simulink model "BESS_Harness"  (R2025b)
settings: Solver=VariableStepAuto  StartTime=0.0  StopTime=5  RelTol=1e-3
PostLoadFcn:
  | BESSParam
values from neighbouring files (symbols this model uses):
  bessVoltage = 1500    [BESSGFLParam.m]    (also in BESSGFMParam.m)
  gflInverter = struct    [BESSGFLParam.m]
  gfmInverter = struct    [BESSGFMParam.m]
  Ts = 5E-5    (= 5e-05)    [BESSGFLParam.m]    (also in BESSGFMParam.m; WindFarmParam.m)
undefined symbols (not defined in the file or in its folder): bessSystem, DiscIntNeverNeededParam, solar
libraries: eeGeneralControl x26, nesl_utility x26, ee_lib x16, simulink x12, fl_lib x10, eeTransforms x7, nesl_utility_internal x4, slpidlib x2, batteryecm_lib x2, simulink_extras x1, eePowerMeasurement x1, eePwmGenerator x1
(part 1 of 4)
settings Model: SimulationMode=accelerator  Creator=skota  LastModifiedBy=skota

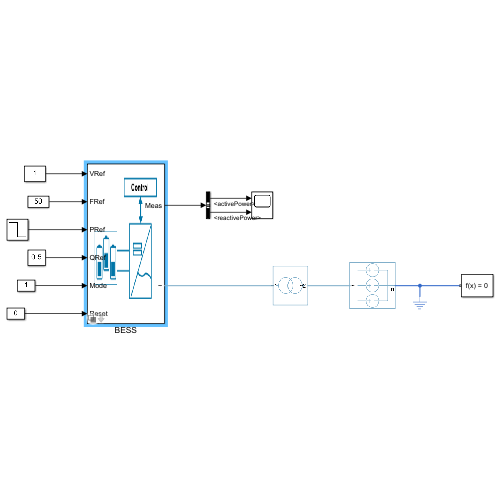
[thumbnail: Simulink's stored preview of the top-level diagram]
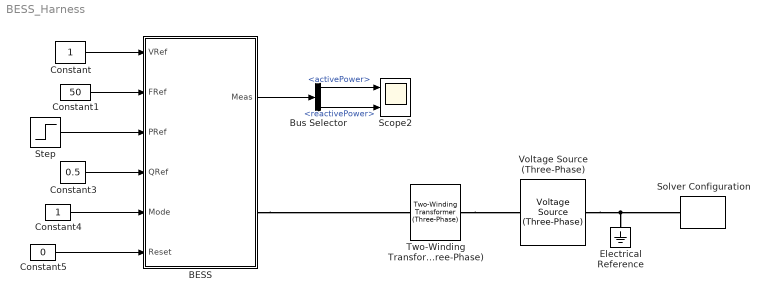
== system BESS_Harness ==
  BESS : Subsystem  Variant=on  VariantControlMode=label  LabelModeActiveChoice=Detailed  mask(Battery Energy Storage System (BESS)){fidelity=Detailed, bessController=Grid Forming, plantRating=bessSystem.plantRating, Vac=bessSystem.Vac, frequency=bessSystem.frequency, iMaxPU=bessSystem.iMaxPU, efficiency=bessSystem.converterEfficiency, baseVoltageDC=bessSystem.Vdc, filterInductance=bessSystem.filterInductance, filterResistance=bessSystem.filterResistance, maxSOC=bessSystem.maxSOC, minSOC=bessSystem.minSOC, converterFidelity=Average, fSw=bessSystem.switchingFrequency, activeDroop=bessSystem.activeDroop, reactiveDroop=bessSystem.reactiveDroop, maxSOCGFM=0.95, minSOCGFM=0.1, initialSOC=0.9, capacityType=Infinite, capacity=1000}
      mask prompts: fidelity "Modeling Option"; bessController "Operating Mode"; plantRating "BESS Rating (kW)"; Vac "Rated AC side voltage (phase-phase RMS) (V)"; frequency "Rated electrical frequency at AC side (Hz)"; iMaxPU "Maximum converter current (pu)"; efficiency "Converter Efficiency (%)"; baseVoltageDC "Voltage on DC side (V)"; filterInductance "Filter inductance (H)"; filterResistance "Filter series resistance (Ohm)"; maxSOC "Maximum  operating SOC"; minSOC "Minimum  operating SOC"; converterFidelity "Converter Fidelity"; fSw "Switching Frequency (kHz)"; activeDroop "Active droop"; reactiveDroop "Reactive droop"; maxSOCGFM "Maximum  operating SOC"; minSOCGFM "Minimum  operating SOC"; initialSOC "Initial SOC"; capacityType "Battery charge capacity"; capacity "Battery capacity (Ah)"
      mask help:
      | This block represents a flexible BESS that can be configured for different operational modes and modeling fidelities. It supports Grid-Following (GFL) and Grid-Forming (GFM) control strategies, along with two fidelity levels:
      |
      | Detailed – captures dynamic control loops and converter behavior for accurate transient analysis.
      | Simplified – optimized for faster simulations while preserving essential system characteristics.
      settings: CopyFcn=set_param(gcbh,'LinkStatus','none');
      mask Help: web('BESS.html')
      mask TypeOptions fidelity: Detailed | Simplified
      mask Callback fidelity:
      | component.mask.fidelitySelection;
      |     fidelity = get_param(gcb,'fidelity');
      |     mode = get_param(gcb,'bessController');
      |     maskObj = Simulink.Mask.get(gcb);
      |     allNames = {maskObj.Parameters.Name};
      |     effIdx = find(strcmp(allNames, 'efficiency'));
      |     tabGFL = maskObj.getDialogControl('cellSimplified');
      |     tabGFM = maskObj.getDialogControl('cellSimplifiedGFM');
      |     if strcmp(fidelity,'Simplified')
      |         maskObj.Parameters(effIdx).Visible = 'on';
      |         if strcmp(mode,'Grid Following')
      |             tabGFL.Visible = 'on';
      |             tabGFM.Visible = 'off';
      |         else
      |             tabGFL.Visible = 'off';
      |             tabGFM.Visible = 'on';
      |         end
      |     else
      |         maskObj.Parameters(effIdx).Visible = 'off';
      |         tabGFL.Visible = 'off';
      |         tabGFM.Visible = 'off';
      |     end
      mask TypeOptions bessController: Grid Following | Grid Forming
      mask Callback bessController:
      | fidelity = get_param(gcb,'fidelity');
      | mode = get_param(gcb,'bessController');
      | if strcmp(fidelity,'Detailed')
      |     component.mask.setBESSController;
      | else
      |     blockPath = [gcb,'/','Simplified'];
      |     component.mask.setBESSController(blockPath);
      | end
      | maskObj = Simulink.Mask.get(gcb);
      | tabGFL = maskObj.getDialogControl('cellSimplified');
      | tabGFM = maskObj.getDialogControl('cellSimplifiedGFM');
      | if strcmp(fidelity,'Simplified')
      |     if strcmp(mode,'Grid Following')
      |         tabGFL.Visible = 'on';
      |         tabGFM.Visible = 'off';
      |     else
      |         tabGFL.Visible = 'off';
      |         tabGFM.Visible = 'on';
      |     end
      | else
      |     tabGFL.Visible = 'off';
      |     tabGFM.Visible = 'off';
      | end
      mask TypeOptions converterFidelity: Detailed/BESS Plant/converterFidelity
      mask Callback converterFidelity:
      | blockPath = [gcb,'/','Detailed','/','BESS Plant','/','Converter'];
      | component.mask.converterFidelity(blockPath);
      mask TypeOptions fSw: Detailed/PV Plant & Controller/PV Plant/fSw
      mask TypeOptions initialSOC: Simplified/Grid Forming/initialSOC
      mask TypeOptions capacityType: Simplified/Grid Forming/capacityType
      mask Callback capacityType: component.mask.configureBatteryCapacity;
      mask TypeOptions capacity: Simplified/Grid Forming/capacity
      mask DialogControl generalDetailed Prompt: General
      mask DialogControl cellDetailed Prompt: Battery
      mask DialogControl configureBattery Prompt: Edit battery parameters
      mask DialogControl configureBattery Callback:
      | blockPath = [gcb,'/','Detailed','/','BESS Plant','/','Battery'] ;
      |     component.mask.openBlock(blockPath);
      mask DialogControl controllerDetailed Prompt: BESS Controller
      mask DialogControl configureBESSController Prompt: Edit BESS Controller
      mask DialogControl configureBESSController Callback:
      | controllerType = get_param(gcb,'bessController');
      |     blockPath = [gcb,'/','Detailed','/','BESS Controller','/',controllerType];
      |     component.mask.openBlock(blockPath);
      mask DialogControl cellSimplified Prompt: Battery
      mask DialogControl configureBatterySimplified Prompt: Edit battery parameters
      mask DialogControl configureBatterySimplified Callback:
      | mode = get_param(gcb,'bessController');
      |     blockPath = [gcb,'/','Simplified','/',mode,'/','Battery'] ;
      |     if strcmp(mode,'Grid Following')
      |         component.mask.openBlock(blockPath);
      |     end
      mask DialogControl converter Prompt: Converter
      mask DialogControl editConverter Prompt: Edit converter parameters
      mask DialogControl editConverter Callback:
      | converterFidelity = get_param(gcb,'converterFidelity');
      | blockPath = [gcb,'/','Detailed','/','BESS Plant','/','Converter','/',converterFidelity,'/','Converter'];
      | component.mask.openBlock(blockPath);
      mask DialogControl cellSimplifiedGFM Prompt: Battery
      mask Display: image('battery_detailed.png');
  Bus Selector : BusSelector  OutputSignals=activePower,reactivePower
  Constant : Constant
  Constant1 : Constant  Value=50
  Constant3 : Constant  Value=0.5
  Constant4 : Constant
  Constant5 : Constant  Value=0
  Electrical Reference : fl_lib/Electrical/Electrical Elements/Electrical Reference
  Scope2 : Scope  NumInputPorts=2
      settings: ActiveDisplayYMinimum=-3.20005915874359  ActiveDisplayYMaximum=1.7817477651289169  DataLoggingVariableName=ScopeData17
  Solver Configuration : nesl_utility/Solver Configuration  PhysicalDomain=network_engine_domain  SubClassName=solver  LeftPortType=input  RightPortType=generic  Tones=[]  Harmonics=[]  SimulateNoise=off  Profile=off  UseLocalSampling=off  EnableSwitchedLinearOptims=on  FrequencyDomain=off  UseCCode=off  RelTol=0.001  AbsTol=0.001  MinStep=1e-09  ToWorkspace=off  RevertToSquareIcSolve=off  NumHomotopyIterations=100  PhasorMode=off  PhasorModeNumHarmonics=1  ConsistencySolver=NEWTON_XTOL_AFTER_FTOL  IndexReductionMethod=DerivativeReplacement  DoDC=off  ResidualTolerance=1e-09  ConsistencyTolSource=GLOBAL  ConsistencyAbsTol=0.001  ConsistencyRelTol=0.001  ConsistencyTolFactor=1e3  UseLocalSolver=on  LocalSolverChoice=NE_BACKWARD_EULER_ADVANCER  ResolveIndetEquations=off  FunctionEvalNumThread=1  LocalSolverSampleTime=5e-5  DoFixedCost=on  MaxNonlinIter=1  MaxModeIter=2  ComputeImpulses=off  ImpulseIterations=2  LinearAlgebra=Sparse  LinearAlgebraNumThread=0  EquationFormulation=NE_TIME_EF  DelaysMemoryBudget=1024  AutomaticFiltering=off  FilteringTimeConstant=0.001  PartitionStorageMethod=AS_NEEDED  PartitionMemoryBudget=1024  PartitionMethod=ROBUST  MultibodyUseLocalSolver=off  MultibodyLocalSolverChoice=ODE1  MultibodyLocalSolverSampleTime=0.001
  Step : Step  Time=30  Before=1  After=0  SampleTime=0
  Two-Winding Transformer (Three-Phase) : ee_lib/Passive/Transformers/Two-Winding Transformer (Three-Phase)  SRated=200e6 A*V  FRated=50 Hz  Winding1Connection=ee.enum.windingconnection.Yg  VRated1=690 V  Winding2Connection=ee.enum.windingconnection.Yg  VRated2=6600 V  CoreType=ee.enum.coretype.threelimb  pu_Rw1=0.01  pu_Rw2=0.01  leakage_reactance_option=ee.enum.transformer_leakage.include  pu_Xl1=0.05  pu_Xl2=0.05  magnetizing_resistance_option=ee.enum.transformer_magnetizingResistance.exclude  pu_Rm=500  magnetizing_reactance_option=ee.enum.transformer_magnetizingReactance.exclude  saturation_option=ee.enum.transformer_saturation.exclude  pu_Xm=500  current_data=[0, .002, 1, 2]  magnetic_flux_data=[0, 1.2, 1.5, 1.51]  pu_X0=0.5  i1_specify=off  i1_priority=None  i1=[0, 0, 0] A  i1_nominal_specify=off  i1_nominal_value=1  i1_nominal_unit=A  i2_specify=off  i2_priority=None  i2=[0, 0, 0] A  i2_nominal_specify=off  i2_nominal_value=1  i2_nominal_unit=A  phi_specify=off  phi_priority=None  phi=[0, 0, 0]  phi_nominal_specify=off  phi_nominal_value=1  phi_nominal_unit=1  power_dissipated_specify=off  power_dissipated_priority=None  power_dissipated=0 W  power_dissipated_nominal_specify=off  power_dissipated_nominal_value=1  power_dissipated_nominal_unit=W
      settings: InternalSimscapePortConfiguration="{\"Bottom\":[],\"Left\":[{\"id\":\"N1\",\"label\":\"~1\",\"type\":\"foundation.electrical.three_phase\"}],\"Right\":[{\"id\":\"N2\",\"label\":\"~2\",\"type\":\"foundation.electrical.three_phase\"}],\"Top\":[]}"
  Voltage Source (Three-Phase) : ee_lib/Sources/Voltage Source (Three-Phase)  vline_rms=6600 V  shift=0 deg  freq=50 Hz  impedance_option=0  SShortCircuit=10e6 A*V  XR=15  R=0.01 Ohm  L=3.97e-4 H  harmonic_option=0  harmonic_orders=[5, 7, 11, 13]  harmonic_ratios=[.1, .1, .1, .1]  G_parasitic=0 1/Ohm  I_specify=off  I_priority=None  I=[0, 0, 0] A  I_nominal_specify=off  I_nominal_value=1  I_nominal_unit=A
  wires:
  Constant/1 -> BESS/1(VRef)
  Constant1/1 -> BESS/2(FRef)
  Constant3/1 -> BESS/4(QRef)
  Constant4/1 -> BESS/5(Mode)
  Constant5/1 -> BESS/6(Reset)
  Step/1 -> BESS/3(PRef)
  BESS/1(Meas) -> Bus Selector/1
  Bus Selector/1 -> Scope2/1  "<activePower>"
  Bus Selector/2 -> Scope2/2  "<reactivePower>"
  connections:
  BESS/RConn1 -- Two-Winding Transformer (Three-Phase)/LConn1
  Two-Winding Transformer (Three-Phase)/RConn1 -- Voltage Source (Three-Phase)/RConn1
  Voltage Source (Three-Phase)/LConn1 -- Solver Configuration/RConn1 -- Electrical Reference/LConn1

== system BESS_Harness/BESS ==
  VRef : Inport
  FRef : Inport  Port=2
  PRef : Inport  Port=3
  QRef : Inport  Port=4
  Mode : Inport  Port=5
  Reset : Inport  Port=6
  Detailed : Subsystem  VariantControl=Detailed
  Simplified : Subsystem  Variant=on  VariantControlMode=label  VariantControl=Simplified  LabelModeActiveChoice=Grid Forming
  ~ : PMIOPort  Side=Right
  Meas : Outport

== system BESS_Harness/BESS/Detailed ==
  note: Plant
  note: Controller
  VRef : Inport
  FRef : Inport  Port=2
  PRef : Inport  Port=3
  QRef : Inport  Port=4
  Mode : Inport  Port=5
  Reset : Inport  Port=6
  BESS Controller : Subsystem  Variant=on  VariantControlMode=label  LabelModeActiveChoice=Grid Forming
  BESS Plant : Subsystem  mask(BESS Plant){converterFidelity=Average, fSw=fSw, ratedVoltage=Vac}
      mask prompts: converterFidelity "Converter Fidelity"; fSw "Switching Frequency (kHz)"; ratedVoltage "Rated voltage on AC side (V)"
      mask help: This block represents the physical interface between the battery and the power converter. It models the electrical and dynamic characteristics of the battery system connected to a converter, while expecting an external control signal for operation
      settings: CopyFcn=set_param(gcbh,'LinkStatus','none');
      mask TypeOptions converterFidelity: Converter/converterFidelity
      mask Callback converterFidelity: component.mask.converterFidelityPlant;
      mask TypeOptions fSw: Converter/fSw
      mask DialogControl Container4 Prompt: General
      mask DialogControl editBattery Prompt: Edit battery parameters
      mask DialogControl editBattery Callback:
      | blockPath = [gcb,'/','Battery'];
      | component.mask.openBlock(blockPath);
      mask DialogControl editConverter Prompt: Edit converter parameters
      mask DialogControl editConverter Callback:
      | converterFidelity = get_param(gcb,'converterFidelity');
      | blockPath = [gcb,'/','Converter','/',converterFidelity,'/','Converter'];
      | component.mask.openBlock(blockPath);
      mask Display: image('battery.png');
  Filter & Measurements : Subsystem
  ~ : PMIOPort  Side=Right
  Meas : Outport
  wires:
  BESS Plant/1(SOC) -> Filter & Measurements/1(SOC)
  FRef/1 -> BESS Controller/2(FRef)
  Mode/1 -> BESS Controller/5(Mode)
  PRef/1 -> BESS Controller/3(PRef)
  Filter & Measurements/1(VIBus) -> BESS Controller/7(VIBus)
  QRef/1 -> BESS Controller/4(QRef)
  VRef/1 -> BESS Controller/1(VRef)
  Reset/1 -> BESS Controller/6(Reset)
  Filter & Measurements/2(Meas) -> Meas/1
  BESS Controller/1(mabc) -> BESS Plant/1(mabc)
  connections:
  Filter & Measurements/RConn1 -- ~/RConn1
  BESS Plant/RConn1 -- Filter & Measurements/LConn1

== system BESS_Harness/BESS/Simplified ==
  VRef : Inport
  FRef : Inport  Port=2
  PRef : Inport  Port=3
  QRef : Inport  Port=4
  Mode : Inport  Port=5
  Reset : Inport  Port=6
  Grid Following : Subsystem  VariantControl=Grid Following  mask(BESS GFL Simplified){plantRating=plantRating, Vac=Vac, frequency=frequency, iMaxPU=iMaxPU, efficiency=efficiency, bessVoltage=baseVoltageDC, maxSOC=maxSOC, minSOC=minSOC}
      mask prompts: plantRating "BESS Rating (kW)"; Vac "Rated AC side voltage (phase-phase RMS) (V)"; frequency "Rated electrical frequency at AC side (Hz)"; iMaxPU "Maximum converter current (pu)"; efficiency "Converter Efficiency (%)"; bessVoltage "Nominal BESS voltage (V)"; maxSOC "Maximum operating SOC"; minSOC "Minimum operating SOC"
      mask help: This block models a BESS that synchronizes with grid voltage and frequency using simplified control representation. This block is designed for computational efficiency, ideal for system-level studies in strong grid conditions where detailed transient behavior is less critical.
      settings: CopyFcn=set_param(gcbh,'LinkStatus','none');
      mask DialogControl generalDetailed Prompt: General
      mask DialogControl Container5 Prompt: Battery
      mask DialogControl editBattery Prompt: Edit battery parameters
      mask DialogControl editBattery Callback:
      | blockPath = [gcb,'/','Battery'] ;
      | component.mask.openBlock(blockPath);
  Grid Forming : Subsystem  VariantControl=Grid Forming  mask(BESS GFM Simplified){plantRating=plantRating, Vac=Vac, frequency=frequency, Vdc=baseVoltageDC, iMaxPU=iMaxPU, efficiency=efficiency, activeDroop=activeDroop, reactiveDroop=reactiveDroop, initialSOC=initialSOC, maxSOC=0.95, minSOC=0.1, capacityType=Infinite, capacity=capacity}
      mask prompts: plantRating "BESS Rating (kW)"; Vac "Rated AC side voltage (phase-phase RMS) (V)"; frequency "Rated electrical frequency at AC side (Hz)"; Vdc "Nominal DC bus voltage (V)"; iMaxPU "Maximum converter current (pu)"; efficiency "Converter Efficiency (%)"; activeDroop "Active droop"; reactiveDroop "Reactive droop"; initialSOC "Initial SOC"; maxSOC "Maximum operating SOC"; minSOC "Minimum operating SOC"; capacityType "Battery charge capacity"; capacity "Battery capacity (Ah)"
      mask help: This block models a BESS with generating voltage and frequency reference capabilities. It is optimized for faster simulations while maintaining essential grid-forming behavior, making it suitable for large-scale stability studies or planning scenarios where detailed converter dynamics are not required.
      settings: CopyFcn=set_param(gcbh,'LinkStatus','none');
      mask TypeOptions capacityType: Fixed | Infinite
      mask Callback capacityType: component.mask.configureBatteryCapacity;
      mask DialogControl generalDetailed Prompt: General
      mask DialogControl Container5 Prompt: Battery
  ~ : PMIOPort  Side=Right
  Meas : Outport

== system BESS_Harness/BESS/Detailed/BESS Controller ==
  VRef : Inport
  FRef : Inport  Port=2
  PRef : Inport  Port=3
  QRef : Inport  Port=4
  Mode : Inport  Port=5
  Reset : Inport  Port=6
  VIBus : Inport  Port=7
  Grid Following : Subsystem  VariantControl=Grid Following  mask(Grid Following Controller){mp=gflInverter.activeDroop, mv=gflInverter.reactiveDroop, P=Real power, MVA=gflInverter.ratedPower, frequency=frequency, zbase=gflInverter.baseImpedance, L=filterInductance%gflInverter.filterInductance, Imax=gflInverter.iMaxPU, Td=gflInverter.sensorDelay, Kpic=gflInverter.kpId, Kiic=gflInverter.kiId, Kd=0}
      mask prompts: mp "Real power droop cofficient"; mv "Reactive power droop cofficient"; P "Priority mode"; MVA "Base Power (V*A)"; frequency "Frequency (Hz)"; zbase "Base Impedance (Ohm)"; L "Filter Inductance (H)"; Imax "Inverter current limit (pu)"; Td "Sensor time delay (s)"; Kpic "Proportional gain"; Kiic "Integral gain"; Kd "Derevative gain"
      mask help: This block implements a Grid Following control strategy where the BESS synchronizes with an existing grid voltage and frequency. Ideal for systems where the grid is strong and the BESS acts as a power source following grid conditions.
      settings: CopyFcn=set_param(gcb,'LinkStatus','none');
      mask TypeOptions P: Real power  | Reactive power
      mask DialogControl Container4 Prompt: General
      mask DialogControl Container5 Prompt: Current Controller
      mask Display: image('gridfollowing2_2_9_7_2_1_1.png');
  Grid Forming : Subsystem  VariantControl=Grid Forming  mask(Grid Forming Controller){power=plantRating*1000, girdLineVoltage=Vac, powerFreq=frequency, dcBusVoltage=bessVoltage, measSampleTime=gfmInverter.measurementSampleTime, powerControl=Virtual Synchronous Machine, activePowerSampleTime=gfmInverter.droopControl.sampleTime, droopSlope=gfmInverter.droopControl.freqSlopeMp*350, droopT1=gfmInverter.droopControl.T1, droopT2=gfmInverter.droopControl.T2, droopTC=gfmInverter.droopControl.lpfTimeConst, vsmPmeasFilterTC=gfmInverter.vsm.PmeasTimeConst, vsmFreqDroop=gfmInverter.vsm.freqDroop, vsmInertiaTC=gfmInverter.vsm.inertiaConstant, vsmDampingConst=gfmInverter.vsm.dampingCoefficent, dampingPowerMaxLimit=gfmInverter.vsm.maxDampingPower, dampingPowerMinLimit=gfmInverter.vsm.minDampingPower, freqMeasTimeConst=gfmInverter.freqMeasTimeConst, freqOption=Constant Frequency Reference, voltreference=gfmInverter.Qcontrol.voltageReference, QVoltFilterTC=gfmInverter.Qcontrol.QmeasTimeConst, QVoltDroop=gfmInverter.Qcontrol.voltageDroop, currentLimit=Current Limiting, maxSatCurrentLimit=gfmInverter.currentLimit.maxSaturationCurrent, maxVICurrentLimit=gfmInverter.currentLimit.viCurrentLimit, ctLimitVirtualImp=gfmInverter.currentLimit.virImpResistanceCoeff, ctLimitXbyR=gfmInverter.currentLimit.virImpXbyR, ctLimitDelayTime=gfmInverter.currentLimit.maxSaturationDelay, currentSatTime=gfmInverter.currentLimit.satCurrentRunTime, currentVITimeConst=gfmInverter.currentLimit.viFilterTimeConst, voltControlTs=gfmInverter.controller.VoltageControlSampleTime, vdPGain=gfmInverter.controller.voltControllerKp, VdIGain=gfmInverter.controller.voltControllerKi, VdMaxCt=gfmInverter.controller.voltageMaxId, VdMinCt=gfmInverter.controller.voltageMinId, VqPGain=gfmInverter.controller.voltControllerKp, VqIGain=gfmInverter.controller.voltControllerKi, VqMaxCt=gfmInverter.controller.voltageMaxIq, VqMinCt=gfmInverter.controller.voltageMinIq, vdvqLPFTimeConst=gfmInverter.controller.voltMeasTimeConst, currentControlTs=gfmInverter.controller.CurrentControlSampleTime, filterInductance=gfmInverter.L, IdPGain=gfmInverter.controller.ctControllerKp, IdIGain=gfmInverter.controller.ctControllerKi, IqPGain=gfmInverter.controller.ctControllerKp, IqIGain=gfmInverter.controller.ctControllerKi}
      mask prompts: power "Grid forming converter power (VA)"; girdLineVoltage "Grid line voltage (V)"; powerFreq "Grid frequency (Hz)"; dcBusVoltage "DC bus voltage"; measSampleTime "Measurement sample time"; powerControl "Active Power Control"; activePowerSampleTime "Sample time (s)"; droopSlope "Power droop slope (pu, Hz/W)"; droopT1 "Lead-Lag numerator time constant (s)"; droopT2 "Lead-Lag denominator time constant (s)"; droopTC "Filter cut-off time constant (s)"; vsmPmeasFilterTC "Power measurement filter time constant (s)"; vsmFreqDroop "Frequency droop (pu,  W/Hz)"; vsmInertiaTC "Inertia constant M (pu)"; vsmDampingConst "Damping constant (pu/Hz)"; dampingPowerMaxLimit "Damping power maximum limit (pu)"; dampingPowerMinLimit "Damping power minimum limit (pu)"; freqMeasTimeConst "Frequency measurement time constant (s)"; freqOption "Damping power fequency option"; voltreference "Voltage reference value (pu)"; QVoltFilterTC "Power measurement filter time constant (s)"; QVoltDroop "Voltage droop (pu, V/VAR)"; currentLimit "Current limiting method"; maxSatCurrentLimit "Maximum current saturation (pu)"; maxVICurrentLimit "Maximum virtual impedance current (pu)"; ctLimitVirtualImp "Virtual impedance coefficient (pu.Ohm/pu.A)"; ctLimitXbyR "Virtual X/R ratio"; ctLimitDelayTime "Maximum current delay time (s)"; currentSatTime "Current limiting run time (s)"; currentVITimeConst "Filter time constant (s)"; voltControlTs "Controller sample time (s)"; vdPGain "Vd proportional gain"; VdIGain "Vd integral gain"; VdMaxCt "Vd maximum current limit (A)"; VdMinCt "Vd minimum current limit (A)"; VqPGain "Vq proportional gain"; VqIGain "Vq integral gain"; VqMaxCt "Vq maximum current limit (A)"; VqMinCt "Vq minimum current limit (A)"; vdvqLPFTimeConst "Voltage measurement filter time constant (s)"; currentControlTs "Controller sample time (s)"; filterInductance "Filter inductance (H)"; IdPGain "Id proportional gain"; IdIGain "Id integral gain"; IqPGain "Iq proportional gain"; IqIGain "Iq integral gain"
      mask help: This block implements the grid forming controller with fault ride through capability. Input to the controller are active and reactive power reference in per unit and the sensed three-phase phase current in amphere and phase voltage in volts.
      mask init:
      | powerChoice = get_param(gcb,'powerControl');
      | currentChoice = get_param(gcb,'currentLimit');
      | 
      | powerloc = [gcb, '/Power Control/ActivePowerControl']; 
      | currentloc = [gcb, '/Current Limiting/CurrentLimitingMethod'];
      | freqLoc = [gcb,'/Power Control/ActivePowerControl/vsmControl/Damping Frequency'];
      | 
      | switch powerChoice
      |     case 'Virtual Synchronous Machine'
      |         set_param(powerloc, 'LabelModeActiveChoice', 'vsm');
      |         dampingFreqChoice = get_param(gcb,'freqOption');
      |         if strcmp(dampingFreqChoice,'Use Grid Frequency Measurement')
      |             set_param(freqLoc, 'LabelModeActiveChoice', 'freqMeas');
      |         else
      |             set_param(freqLoc, 'LabelModeActiveChoice', 'constFreq');
      |         end
      |     case 'Droop Control'
      |          set_param(powerloc, 'LabelModeActiveChoice', 'droop');
      |    otherwise
      |         disp('Choose proper active power control method')
      | end
      | switch currentChoice
      |     case 'Virtual Impedance'
      |           set_param(currentloc, 'LabelModeActiveChoice', 'virimp');
      |     case 'Current Limiting'
      |          set_param(currentloc, 'LabelModeActiveChoice', 'ctSat');
      |     case 'Combining Virtual Impedance and Current Limiting'
      |             set_param(currentloc, 'LabelModeActiveChoice', 'both');
      |     otherwise
      |         disp('Choose proper current limiting method')
      | end
      settings: CopyFcn=set_param(gcb,'LinkStatus','none');
      mask TypeOptions powerControl: Virtual Synchronous Machine | Droop Control
      mask Callback powerControl:
      | h = Simulink.Mask.get(gcb);
      | slectedActivePowerControl=get_param(gcb,'powerControl');
      | %slectedActivePowerControl = h.Parameters(find(string({h.Parameters.Name}) == 'powerControl')).Value;
      | switch slectedActivePowerControl
      |     case 'Virtual Synchronous Machine'
      |         h.Parameters(find(string({h.Parameters.Name}) == 'droopSlope')).Visible = 'off';
      |         h.Parameters(find(string({h.Parameters.Name}) == 'droopTC')).Visible = 'off';
      |         h.Parameters(find(string({h.Parameters.Name}) == 'droopT1')).Visible = 'off';
      |         h.Parameters(find(string({h.Parameters.Name}) == 'droopT2')).Visible = 'off';
      |         h.Parameters(find(string({h.Parameters.Name}) == 'vsmPmeasFilterTC')).Visible = 'on';
      |         h.Parameters(find(string({h.Parameters.Name}) == 'vsmFreqDroop')).Visible = 'on';
      |         h.Parameters(find(string({h.Parameters.Name}) == 'vsmInertiaTC')).Visible = 'on';
      |         h.Parameters(find(string({h.Parameters.Name}) == 'vsmDampingConst')).Visible = 'on';
      |         h.Parameters(find(string({h.Parameters.Name}) == 'dampingPowerMaxLimit')).Visible = 'on';
      |         h.Parameters(find(string({h.Parameters.Name}) == 'dampingPowerMinLimit')).Visible = 'on';
      |         h.Parameters(find(string({h.Parameters.Name}) == 'freqOption')).Visible = 'on';
      |         h.Parameters(find(string({h.Parameters.Name}) == 'freqMeasTimeConst')).Visible = 'on';
      |     case 'Droop Control'
      |         h.Parameters(find(string({h.Parameters.Name}) == 'droopSlope')).Visible = 'on';
      |         h.Parameters(find(string({h.Parameters.Name}) == 'droopTC')).Visible = 'on';
      |         h.Parameters(find(string({h.Parameters.Name}) == 'droopT1')).Visible = 'on';
      |         h.Parameters(find(string({h.Parameters.Name}) == 'droopT2')).Visible = 'on';
      |         h.Parameters(find(string({h.Parameters.Name}) == 'vsmPmeasFilterTC')).Visible = 'off';
      |         h.Parameters(find(string({h.Parameters.Name}) == 'vsmFreqDroop')).Visible = 'off';
      |         h.Parameters(find(string({h.Parameters.Name}) == 'vsmInertiaTC')).Visible = 'off';
      |         h.Parameters(find(string({h.Parameters.Name}) == 'vsmDampingConst')).Visible = 'off';
      |         h.Parameters(find(string({h.Parameters.Name}) == 'dampingPowerMaxLimit')).Visible = 'off';
      |         h.Parameters(find(string({h.Parameters.Name}) == 'dampingPowerMinLimit')).Visible = 'off';
      |         h.Parameters(find(string({h.Parameters.Name}) == 'freqOption')).Visible = 'off';
      |         h.Parameters(find(string({h.Parameters.Name}) == 'freqMeasTimeConst')).Visible = 'on';
      | 
      |     otherwise
      |         disp('Choose proper active power control method')
      | end
      mask TypeOptions freqOption: Use Grid Frequency Measurement | Constant Frequency Reference
      mask TypeOptions currentLimit: Virtual Impedance | Current Limiting | Combining Virtual Impedance and Current Limiting
      mask Callback currentLimit:
      | currentLimit = 1;
      | h = Simulink.Mask.get(gcb);
      | currentLimitControl=get_param(gcb,'currentLimit');
      | %slectedActivePowerControl = h.Parameters(find(string({h.Parameters.Name}) == 'powerControl')).Value;
      | switch currentLimitControl
      |     case 'Virtual Impedance'
      |         h.Parameters(find(string({h.Parameters.Name}) == 'maxVICurrentLimit')).Visible = 'on';
      |         h.Parameters(find(string({h.Parameters.Name}) == 'ctLimitVirtualImp')).Visible = 'on';
      |         h.Parameters(find(string({h.Parameters.Name}) == 'ctLimitXbyR')).Visible = 'on';
      |         h.Parameters(find(string({h.Parameters.Name}) == 'maxSatCurrentLimit')).Visible = 'off';
      |         h.Parameters(find(string({h.Parameters.Name}) == 'ctLimitDelayTime')).Visible = 'off';
      |         h.Parameters(find(string({h.Parameters.Name}) == 'currentSatTime')).Visible = 'off';
      |         h.Parameters(find(string({h.Parameters.Name}) == 'currentVITimeConst')).Visible = 'on';
      | 
      | 
      |     case 'Current Limiting'
      |         h.Parameters(find(string({h.Parameters.Name}) == 'maxVICurrentLimit')).Visible = 'off';
      |         h.Parameters(find(string({h.Parameters.Name}) == 'ctLimitVirtualImp')).Visible = 'off';
      |         h.Parameters(find(string({h.Parameters.Name}) == 'ctLimitXbyR')).Visible = 'off';
      |         h.Parameters(find(string({h.Parameters.Name}) == 'maxSatCurrentLimit')).Visible = 'on';
      |         h.Parameters(find(string({h.Parameters.Name}) == 'ctLimitDelayTime')).Visible = 'on';
      |         h.Parameters(find(string({h.Parameters.Name}) == 'currentSatTime')).Visible = 'off';
      |         h.Parameters(find(string({h.Parameters.Name}) == 'currentVITimeConst')).Visible = 'off';
      | 
      |     case 'Combining Virtual Impedance and Current Limiting'
      |         h.Parameters(find(string({h.Parameters.Name}) == 'maxVICurrentLimit')).Visible = 'on';
      |         h.Parameters(find(string({h.Parameters.Name}) == 'ctLimitVirtualImp')).Visible = 'on';
      |         h.Parameters(find(string({h.Parameters.Name}) == 'ctLimitXbyR')).Visible = 'on';
      |         h.Parameters(find(string({h.Parameters.Name}) == 'maxSatCurrentLimit')).Visible = 'on';
      |         h.Parameters(find(string({h.Parameters.Name}) == 'ctLimitDelayTime')).Visible = 'off';
      |         h.Parameters(find(string({h.Parameters.Name}) == 'currentSatTime')).Visible = 'on';
      |         h.Parameters(find(string({h.Parameters.Name}) == 'currentVITimeConst')).Visible = 'on';
      | 
      |     otherwise
      |         disp('Choose proper current limiting method')
      | end
      mask DialogControl ParameterGroupVar Prompt: Grid Forming Control Parameters
      mask DialogControl Container8 Prompt: Grid-forming Converter Specification
      mask DialogControl Pcontrolgrp Prompt: Active Power Controller Parameters
      mask DialogControl QcontrolGrp Prompt: Reactive Power Controller Parameters
      mask DialogControl faultRideThroughGrp Prompt: Fault Ride Through Parameters
      mask DialogControl voltControlgrp Prompt: Voltage Controller Parameters
      mask DialogControl Container15currentContGrp Prompt: Current Controller Parameters
      mask Display: image('gfmGridFormingConverterVSM1_1_7_7_2.png');
  mabc : Outport

== system BESS_Harness/BESS/Detailed/BESS Plant ==
  mabc : Inport
  Battery : batteryecm_lib/Battery  Vnom=bessVoltage V  prm_dir=simscape.enum.battery.prm_dir.disabled  R1_dis=2 Ohm  R1_ch=2 Ohm  R1=0.001 Ohm  prm_AH=simscape.enum.battery.prm_AH.infinite  AH=50 A*hr  V1=11.5 V  AH1=25 A*hr  prm_R2=simscape.enum.battery.prm_R2.disabled  R2=2000 Ohm  Tmeas=298.15 K  charge_measurement_port=simscape.enum.battery.enable.yes  prm_dyn=simscape.enum.battery.prm_dyn.off  Rp1=0.005 Ohm  tau1=30 s  Rp2=0.005 Ohm  tau2=30 s  Rp3=0.005 Ohm  tau3=30 s  Rp4=0.005 Ohm  tau4=30 s  Rp5=0.005 Ohm  tau5=30 s  prm_fade=simscape.enum.battery.prm_fade.disabled  N_fade=100  AH_fade=45 A*hr  R1_fade=2.02 Ohm  R1_ch_fade=2.02 Ohm  V1_fade=10.35 V  prm_age=simscape.enum.battery.prm_age.disabled  prm_age_OCV=simscape.enum.battery.prm_age_OCV.OCV  OCV_age=0.9  SOC_age=60  Tmeas_age=298.15 K  delta_time_age_vec=[0] d  temperature_age_vec=[273] K  OCV_scaling_age=2.2134e6  OCV_offset_age=1.632e6  temp_exp_age=0.515833569 V  t_exp_age=0.75  Vnom_T2=12 V  R1_T2=2.2 Ohm  R1_T2_dis=2.2 Ohm  R1_T2_ch=2.2 Ohm  V1_T2=11.4 V  R2_T2=2200 Ohm  Rp1_T2=0.005 Ohm  tau1_T2=30 s  Rp2_T2=0.005 Ohm  tau2_T2=30 s  Rp3_T2=0.005 Ohm  tau3_T2=30 s  Rp4_T2=0.005 Ohm  tau4_T2=30 s  Rp5_T2=0.005 Ohm  tau5_T2=30 s  Tmeas2=273.15 K  thermal_port=simscape.enum.thermaleffects.omit  thermal_mass=30000 J/K  i_specify=off  i_priority=None  i=0 A  i_nominal_specify=off  i_nominal_value=1  i_nominal_unit=A  v_specify=off  v_priority=None  v=0 V  v_nominal_specify=off  v_nominal_value=1  v_nominal_unit=V  charge_specify=off  charge_priority=High  charge=50 A*hr  charge_nominal_specify=off  charge_nominal_value=1  charge_nominal_unit=A*hr  num_cycles_specify=off  num_cycles_priority=High  num_cycles=0  num_cycles_nominal_specify=off  num_cycles_nominal_value=1  num_cycles_nominal_unit=1  temperature_specify=off  temperature_priority=High  temperature=298.15 K  temperature_nominal_specify=off  temperature_nominal_value=1  temperature_nominal_unit=K
      settings: InternalSimscapePortConfiguration="{\"Bottom\":[],\"Left\":[{\"id\":\"p\",\"label\":\"+\",\"type\":\"foundation.electrical.electrical\"},{\"id\":\"q\",\"label\":\"q\",\"type\":\"output\"}],\"Right\":[{\"id\":\"n\",\"label\":\"-\",\"type\":\"foundation.electrical.electrical\"}],\"Top\":[]}"
  Converter : Subsystem  InitFcn=%solar.mask.restoreConverterLink(gcb);  Variant=on  VariantControlMode=label  LabelModeActiveChoice=Average  mask{converterFidelity=Average, fSw=fSw}
      mask prompts: converterFidelity "Converter Fidelity"; fSw "Switching Frequency (kHz)"
      settings: PreSaveFcn=%solar.mask.restoreConverterLink  CloseFcn=%solar.mask.restoreConverterLink
      mask TypeOptions converterFidelity: Average | Switching
      mask Callback converterFidelity: component.mask.converterFidelity(gcb);
      mask DialogControl editSwitch Prompt: Edit converter parameters
      mask DialogControl editSwitch Callback:
      | converterFidelity = get_param(gcb,'converterFidelity');
      | blockPath = [gcb,'/',converterFidelity,'/','Converter'];
      | component.mask.openBlock(blockPath);
  Electrical Reference1 : fl_lib/Electrical/Electrical Elements/Electrical Reference
  PS-Simulink Converter : nesl_utility/PS-Simulink Converter  PhysicalDomain=network_engine_domain  SubClassName=ps_output  LeftPortType=input  RightPortType=output  PseudoPeriodic=off  Frequencies=[]  VectorFormat=inherit  Unit=inherit  AffineConversion=off
  ~ : PMIOPort  Side=Right
  SOC : Outport
  wires:
  PS-Simulink Converter/1 -> SOC/1
  mabc/1 -> Converter/1(mabc)
  connections:
  PS-Simulink Converter/LConn1 -- Battery/LConn2
  ~/RConn1 -- Converter/RConn1
  Battery/LConn1 -- Converter/LConn1
  Converter/LConn2 -- Electrical Reference1/LConn1 -- Battery/RConn1

== system BESS_Harness/BESS/Detailed/Filter & Measurements ==
  SOC : Inport
  Current and Voltage Sensor (Three-Phase) : ee_lib/Sensors & Transducers/Current and Voltage Sensor (Three-Phase)  vMeasurementType=ee.enum.vmeasurement.lg  outputUnit=ee.enum.unit.pu  SRated=plantRating*1000 A*V  VRated=Vac V  I_specify=off  I_priority=None  I=[ 0 0 0 ] A  I_nominal_specify=off  I_nominal_value=1  I_nominal_unit=A  V_specify=off  V_priority=None  V=[ 0 0 0 ] V  V_nominal_specify=off  V_nominal_value=1  V_nominal_unit=V
      settings: InternalSimscapePortConfiguration="{\"Bottom\":[],\"Left\":[{\"id\":\"N1\",\"label\":\"~1\",\"type\":\"foundation.electrical.three_phase\"}],\"Right\":[{\"id\":\"V_output\",\"label\":\"V\",\"type\":\"output\"},{\"id\":\"I_output\",\"label\":\"I\",\"type\":\"output\"},{\"id\":\"N2\",\"label\":\"~2\",\"type\":\"foundation.electrical.three_phase\"}],\"Top\":[]}"
  Gain : Gain  Gain=1/(plantRating*1000)
  Gain1 : Gain  Gain=1/(plantRating*1000)
  Low-Pass Filter (Discrete or Continuous) : eeGeneralControl/Low-Pass Filter (Discrete or Continuous)  K=1  T=0.02  B=inf  A=-inf  init_option=Inherited from block input  x0=0  Ts=Ts
  Low-Pass Filter (Discrete or Continuous)1 : eeGeneralControl/Low-Pass Filter (Discrete or Continuous)  K=1  T=0.02  B=inf  A=-inf  init_option=Inherited from block input  x0=0  Ts=Ts
  PLL & Measurements : Subsystem
      mask Display: image('PLL_9_7_2.png');
  PS-Simulink Converter2 : nesl_utility_internal/PS-Simulink Converter  PhysicalDomain=network_engine_domain  SubClassName=ps_output  LeftPortType=input  RightPortType=output  PseudoPeriodic=off  Frequencies=[]  VectorFormat=1-D array  Unit=V  AffineConversion=off
  PS-Simulink Converter3 : nesl_utility_internal/PS-Simulink Converter  PhysicalDomain=network_engine_domain  SubClassName=ps_output  LeftPortType=input  RightPortType=output  PseudoPeriodic=off  Frequencies=[]  VectorFormat=1-D array  Unit=A  AffineConversion=off
  PS-Simulink Converter6 : nesl_utility_internal/PS-Simulink Converter  PhysicalDomain=network_engine_domain  SubClassName=ps_output  LeftPortType=input  RightPortType=output  PseudoPeriodic=off  Frequencies=[]  VectorFormat=1-D array  Unit=W  AffineConversion=off
  PS-Simulink Converter7 : nesl_utility_internal/PS-Simulink Converter  PhysicalDomain=network_engine_domain  SubClassName=ps_output  LeftPortType=input  RightPortType=output  PseudoPeriodic=off  Frequencies=[]  VectorFormat=1-D array  Unit=V*A  AffineConversion=off
  Power Sensor (Three-Phase)1 : ee_lib/Sensors & Transducers/Power Sensor (Three-Phase)  load_type=ee.enum.passive.type_balanced.balanced  f0=60 Hz
      settings: InternalSimscapePortConfiguration="{\"Bottom\":[],\"Left\":[{\"id\":\"N1\",\"label\":\"~1\",\"type\":\"foundation.electrical.three_phase\"}],\"Right\":[{\"id\":\"N2\",\"label\":\"~2\",\"type\":\"foundation.electrical.three_phase\"}],\"Top\":[{\"id\":\"Pm\",\"label\":\"P\",\"type\":\"output\"},{\"id\":\"Qm\",\"label\":\"Q\",\"type\":\"output\"}]}"
  RLC (Three-Phase) : ee_lib/Passive/RLC Assemblies/RLC (Three-Phase)  port_option=ee.enum.threePhasePort.composite  component_structure=ee.enum.rlc.structure.SeriesRL  R=gfmInverter.lineResistance Ohm  L=gfmInverter.L H  C=1e-6 F  R_parasitic=0 Ohm  G_parasitic=0 1/Ohm  IL_specify=on  IL_priority=None  IL=[0, 0, 0] A  IL_nominal_specify=off  IL_nominal_value=1  IL_nominal_unit=A  VC_specify=off  VC_priority=High  VC=[0, 0, 0] V  VC_nominal_specify=off  VC_nominal_value=1  VC_nominal_unit=V
      settings: InternalSimscapePortConfiguration="{\"Bottom\":[],\"Left\":[{\"id\":\"N1\",\"label\":\"~1\",\"type\":\"foundation.electrical.three_phase\"}],\"Right\":[{\"id\":\"N2\",\"label\":\"~2\",\"type\":\"foundation.electrical.three_phase\"}],\"Top\":[]}"
  In : PMIOPort  Side=Left
  ~ : PMIOPort  Port=2  Side=Right
  VIBus : Outport
  Out Bus Element : Outport  Port=2  PortName=Meas  Element=voltage
  Out Bus Element1 : Outport  Port=2  PortName=Meas  Element=current
  Out Bus Element2 : Outport  Port=2  PortName=Meas  Element=activePower
  Out Bus Element3 : Outport  Port=2  PortName=Meas  Element=reactivePower
  BusElementOut : Outport  Port=2  PortName=Meas  Element=SOC
  wires:
  SOC/1 -> BusElementOut/1
  Gain1/1 -> Out Bus Element3/1
  Gain/1 -> Out Bus Element2/1
  PS-Simulink Converter2/1 -> Out Bus Element/1, PLL & Measurements/1(V)
  PS-Simulink Converter6/1 -> Low-Pass Filter (Discrete or Continuous)1/1
  PS-Simulink Converter7/1 -> Low-Pass Filter (Discrete or Continuous)/1
  PS-Simulink Converter3/1 -> Out Bus Element1/1, PLL & Measurements/2(I)
  Low-Pass Filter (Discrete or Continuous)/1 -> Gain1/1
  Low-Pass Filter (Discrete or Continuous)1/1 -> Gain/1
  PLL & Measurements/1(VIbus) -> VIBus/1
  connections:
  Power Sensor (Three-Phase)1/LConn1 -- Current and Voltage Sensor (Three-Phase)/RConn3
  PS-Simulink Converter2/LConn1 -- Current and Voltage Sensor (Three-Phase)/RConn1
  Current and Voltage Sensor (Three-Phase)/RConn2 -- PS-Simulink Converter3/LConn1
  Power Sensor (Three-Phase)1/LConn2 -- PS-Simulink Converter6/LConn1
  Power Sensor (Three-Phase)1/LConn3 -- PS-Simulink Converter7/LConn1
  RLC (Three-Phase)/RConn1 -- Current and Voltage Sensor (Three-Phase)/LConn1
  Power Sensor (Three-Phase)1/RConn1 -- ~/RConn1
  In/RConn1 -- RLC (Three-Phase)/LConn1

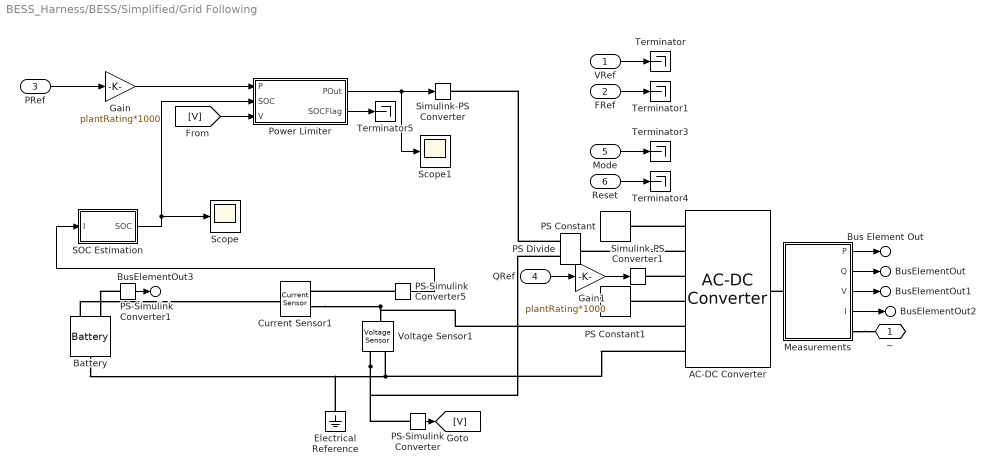
== system BESS_Harness/BESS/Simplified/Grid Following ==
  VRef : Inport
  FRef : Inport  Port=2
  PRef : Inport  Port=3
  QRef : Inport  Port=4
  Mode : Inport  Port=5
  Reset : Inport  Port=6
  AC-DC Converter : custom_lib/AC-DC Converter  port_option=ee.enum.threePhasePort.composite  FRated=frequency Hz  Vline_rms_ini=Vac/4 V  VRated=Vac V  Vang_ini=0 deg  IMaxPU=iMaxPU  PRated=plantRating kW  efficiency=efficiency
      settings: InternalSimscapePortConfiguration="{\"Bottom\":[],\"Left\":[{\"id\":\"Vref\",\"label\":\"Vref\",\"type\":\"input\"},{\"id\":\"Iref\",\"label\":\"Iref\",\"type\":\"input\"},{\"id\":\"Qref\",\"label\":\"Qref\",\"type\":\"input\"},{\"id\":\"Mode\",\"label\":\"Mode\",\"type\":\"input\"},{\"id\":\"p\",\"label\":\"+\",\"type\":\"foundation.electrical.electrical\"},{\"id\":\"n\",\"label\":\"-\",\"type\":\"foundation.electrical.electrical\"}],\"Right\":[{\"id\":\"N\",\"label\":\"~\",\"type\":\"foundation.electrical.three_phase\"}],\"Top\":[]}"
  Battery : batteryecm_lib/Battery  Vnom=bessVoltage V  prm_dir=simscape.enum.battery.prm_dir.disabled  R1_dis=2 Ohm  R1_ch=2 Ohm  R1=1e-3 Ohm  prm_AH=simscape.enum.battery.prm_AH.infinite  AH=50 A*hr  V1=11.5 V  AH1=25 A*hr  prm_R2=simscape.enum.battery.prm_R2.disabled  R2=2000 Ohm  Tmeas=298.15 K  charge_measurement_port=simscape.enum.battery.enable.yes  prm_dyn=simscape.enum.battery.prm_dyn.off  Rp1=0.005 Ohm  tau1=30 s  Rp2=0.005 Ohm  tau2=30 s  Rp3=0.005 Ohm  tau3=30 s  Rp4=0.005 Ohm  tau4=30 s  Rp5=0.005 Ohm  tau5=30 s  prm_fade=simscape.enum.battery.prm_fade.disabled  N_fade=100  AH_fade=45 A*hr  R1_fade=2.02 Ohm  R1_ch_fade=2.02 Ohm  V1_fade=10.35 V  prm_age=simscape.enum.battery.prm_age.disabled  prm_age_OCV=simscape.enum.battery.prm_age_OCV.OCV  OCV_age=0.9  SOC_age=60  Tmeas_age=298.15 K  delta_time_age_vec=[0] d  temperature_age_vec=[273] K  OCV_scaling_age=2.2134e6  OCV_offset_age=1.632e6  temp_exp_age=0.515833569 V  t_exp_age=0.75  Vnom_T2=12 V  R1_T2=2.2 Ohm  R1_T2_dis=2.2 Ohm  R1_T2_ch=2.2 Ohm  V1_T2=11.4 V  R2_T2=2200 Ohm  Rp1_T2=0.005 Ohm  tau1_T2=30 s  Rp2_T2=0.005 Ohm  tau2_T2=30 s  Rp3_T2=0.005 Ohm  tau3_T2=30 s  Rp4_T2=0.005 Ohm  tau4_T2=30 s  Rp5_T2=0.005 Ohm  tau5_T2=30 s  Tmeas2=273.15 K  thermal_port=simscape.enum.thermaleffects.omit  thermal_mass=30000 J/K  i_specify=off  i_priority=None  i=0 A  i_nominal_specify=off  i_nominal_value=1  i_nominal_unit=A  v_specify=off  v_priority=None  v=0 V  v_nominal_specify=off  v_nominal_value=1  v_nominal_unit=V  charge_specify=off  charge_priority=High  charge=50 A*hr  charge_nominal_specify=off  charge_nominal_value=1  charge_nominal_unit=A*hr  num_cycles_specify=off  num_cycles_priority=High  num_cycles=0  num_cycles_nominal_specify=off  num_cycles_nominal_value=1  num_cycles_nominal_unit=1  temperature_specify=off  temperature_priority=High  temperature=298.15 K  temperature_nominal_specify=off  temperature_nominal_value=1  temperature_nominal_unit=K
      settings: InternalSimscapePortConfiguration="{\"Bottom\":[],\"Left\":[{\"id\":\"p\",\"label\":\"+\",\"type\":\"foundation.electrical.electrical\"},{\"id\":\"q\",\"label\":\"q\",\"type\":\"output\"}],\"Right\":[{\"id\":\"n\",\"label\":\"-\",\"type\":\"foundation.electrical.electrical\"}],\"Top\":[]}"
  Current Sensor1 : fl_lib/Electrical/Electrical Sensors/Current Sensor
  Electrical Reference : fl_lib/Electrical/Electrical Elements/Electrical Reference
  Gain : Gain  Gain=plantRating*1000
  Gain1 : Gain  Gain=plantRating*1000
  Measurements : Subsystem
  PS Constant : fl_lib/Physical Signals/Sources/PS Constant  constant=0
  PS Constant1 : fl_lib/Physical Signals/Sources/PS Constant  constant=1
  PS Divide : fl_lib/Physical Signals/Functions/PS Divide
  PS-Simulink Converter : nesl_utility/PS-Simulink Converter  PhysicalDomain=network_engine_domain  SubClassName=ps_output  LeftPortType=input  RightPortType=output  PseudoPeriodic=off  Frequencies=[]  VectorFormat=inherit  Unit=inherit  AffineConversion=off
  PS-Simulink Converter1 : nesl_utility/PS-Simulink Converter  PhysicalDomain=network_engine_domain  SubClassName=ps_output  LeftPortType=input  RightPortType=output  PseudoPeriodic=off  Frequencies=[]  VectorFormat=inherit  Unit=inherit  AffineConversion=off
  PS-Simulink Converter5 : nesl_utility/PS-Simulink Converter  PhysicalDomain=network_engine_domain  SubClassName=ps_output  LeftPortType=input  RightPortType=output  PseudoPeriodic=off  Frequencies=[]  VectorFormat=inherit  Unit=inherit  AffineConversion=off
  Power Limiter : Subsystem
  SOC Estimation : Subsystem
  Scope : Scope
      settings: ActiveDisplayYMinimum=-1  ActiveDisplayYMaximum=1  DataLoggingVariableName=ScopeData21
  Scope1 : Scope
  Simulink-PS Converter : nesl_utility/Simulink-PS Converter  PhysicalDomain=network_engine_domain  SubClassName=ps_input  LeftPortType=input  RightPortType=output  PseudoPeriodic=off  Frequencies=[]  NoiseDistribution=none  NoiseParameters=[]  Unit=V*A  AffineConversion=off  FilteringAndDerivatives=provide  SimscapeFilterOrder=1  InputFilterTimeConstant=0.001  UdotUserProvided=0
  Simulink-PS Converter1 : nesl_utility/Simulink-PS Converter  PhysicalDomain=network_engine_domain  SubClassName=ps_input  LeftPortType=input  RightPortType=output  PseudoPeriodic=off  Frequencies=[]  NoiseDistribution=none  NoiseParameters=[]  Unit=1  AffineConversion=off  FilteringAndDerivatives=provide  SimscapeFilterOrder=1  InputFilterTimeConstant=0.001  UdotUserProvided=0
  Terminator{,1,3..5} (5 alike) : Terminator
  Voltage Sensor1 : fl_lib/Electrical/Electrical Sensors/Voltage Sensor
  ~ : PMIOPort  Side=Right
  Bus Element Out : Outport  PortName=Meas  Element=activePower
  BusElementOut : Outport  PortName=Meas  Element=reactivePower
  BusElementOut1 : Outport  PortName=Meas  Element=voltage
  BusElementOut2 : Outport  PortName=Meas  Element=current
  BusElementOut3 : Outport  PortName=Meas  Element=SOC
  wires:
  PS-Simulink Converter1/1 -> BusElementOut3/1
  Measurements/4(I) -> BusElementOut2/1
  Measurements/2(Q) -> BusElementOut/1
  Measurements/3(V) -> BusElementOut1/1
  Measurements/1(P) -> Bus Element Out/1
  Gain1/1 -> Simulink-PS Converter1/1
  PRef/1 -> Gain/1
  Power Limiter/2(SOCFlag) -> Terminator5/1
  Power Limiter/1(POut) -> Scope1/1, Simulink-PS Converter/1
  Reset/1 -> Terminator4/1
  SOC Estimation/1(SOC) -> Scope/1, Power Limiter/2(SOC)
  [V] -> Power Limiter/3(V)
  Mode/1 -> Terminator3/1
  PS-Simulink Converter5/1 -> SOC Estimation/1(I)
  QRef/1 -> Gain1/1
  FRef/1 -> Terminator1/1
  VRef/1 -> Terminator/1
  PS-Simulink Converter/1 -> [V]
  Gain/1 -> Power Limiter/1(P)
  connections:
  PS-Simulink Converter1/LConn1 -- Battery/LConn2
  Measurements/RConn1 -- ~/RConn1
  Measurements/LConn1 -- AC-DC Converter/RConn1
  AC-DC Converter/LConn3 -- Simulink-PS Converter1/RConn1
  AC-DC Converter/LConn1 -- PS Constant/RConn1
  Battery/LConn1 -- Current Sensor1/LConn1
  PS Divide/LConn1 -- Simulink-PS Converter/RConn1
  PS-Simulink Converter5/LConn1 -- Current Sensor1/RConn1
  AC-DC Converter/LConn2 -- PS Divide/RConn1
  AC-DC Converter/LConn4 -- PS Constant1/RConn1
  AC-DC Converter/LConn5 -- Voltage Sensor1/LConn1 -- Current Sensor1/RConn2
  AC-DC Converter/LConn6 -- Voltage Sensor1/RConn2 -- Electrical Reference/LConn1 -- Battery/RConn1
  Voltage Sensor1/RConn1 -- PS-Simulink Converter/LConn1 -- PS Divide/LConn2
